simulink model "Assignment1_1"  (R2023a)
settings: Solver=VariableStepAuto  StartTime=0.0  StopTime=10  RelTol=1e-3
settings Model: Creator=nicos  LastModifiedBy=nicos

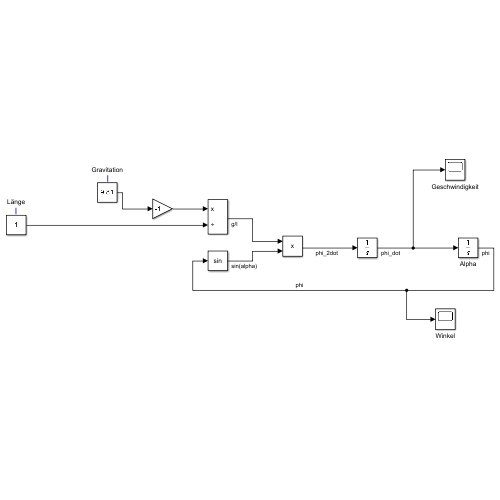
[thumbnail: Simulink's stored preview of the top-level diagram]
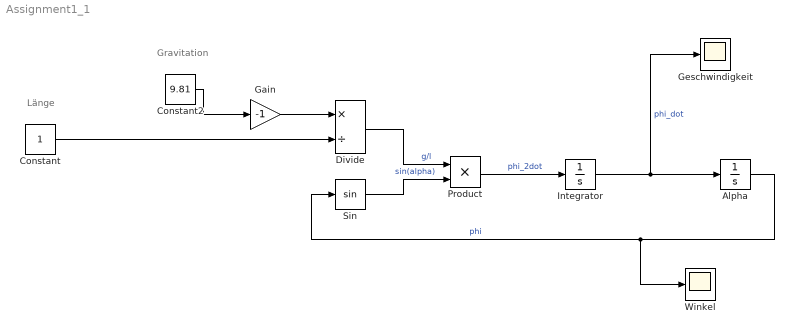
== system Assignment1_1 ==
  note: Gravitation
  note: Länge
  Alpha : Integrator  InitialCondition=30
  Constant : Constant
  Constant2 : Constant  Value=9.81
  Divide : Product  Inputs=*/
  Gain : Gain  Gain=-1
  Geschwindigkeit : Scope
  Integrator : Integrator
  Product : Product
  Sin : Trigonometry
  Winkel : Scope
  wires:
  Constant2/1 -> Gain/1
  Constant/1 -> Divide/2
  Alpha/1 -> Winkel/1, Sin/1  "phi"
  Gain/1 -> Divide/1
  Sin/1 -> Product/2  "sin(alpha)"
  Divide/1 -> Product/1  "g/l"
  Integrator/1 -> Geschwindigkeit/1, Alpha/1  "phi_dot"
  Product/1 -> Integrator/1  "phi_2dot"
